simulink model "leg"  (R2014a)
settings: Solver=FixedStepDiscrete  StartTime=0.0  StopTime=inf  FixedStep=0.001  RelTol=1e-3
libraries: xpcethercatlib x35, simulink x29, slrtlib x11
settings Model: xpc_rtwmakecfg_data=_xpcethercatlib_  SimulationMode=external  BufferReuse=off  Creator=drl  LastModifiedBy=drl
settings SolverCC: EnableConcurrentExecution=on  ConcurrentTasks=on
settings OptimizationCC: BlockReduction=off  OptimizeBlockIOStorage=off  BufferReuse=off  GlobalBufferReuse=off  ExpressionFolding=off  LocalBlockOutputs=off
settings HardwareCC: ProdIntDivRoundTo=Zero  ProdEndianess=LittleEndian  ProdHWDeviceType=Generic->32-bit x86 compatible
settings RTWCC: SystemTargetFile=slrt.tlc  TemplateMakefile=slrt_default_tmf  Description=Simulink Real-Time  ProcessScript=slrt_make_rtw_hook  RTWCompilerOptimization=On
settings SimulinkRealTimeCC: GeneratePreprocessorConditionals=Disable all  EnableShiftOperators=on

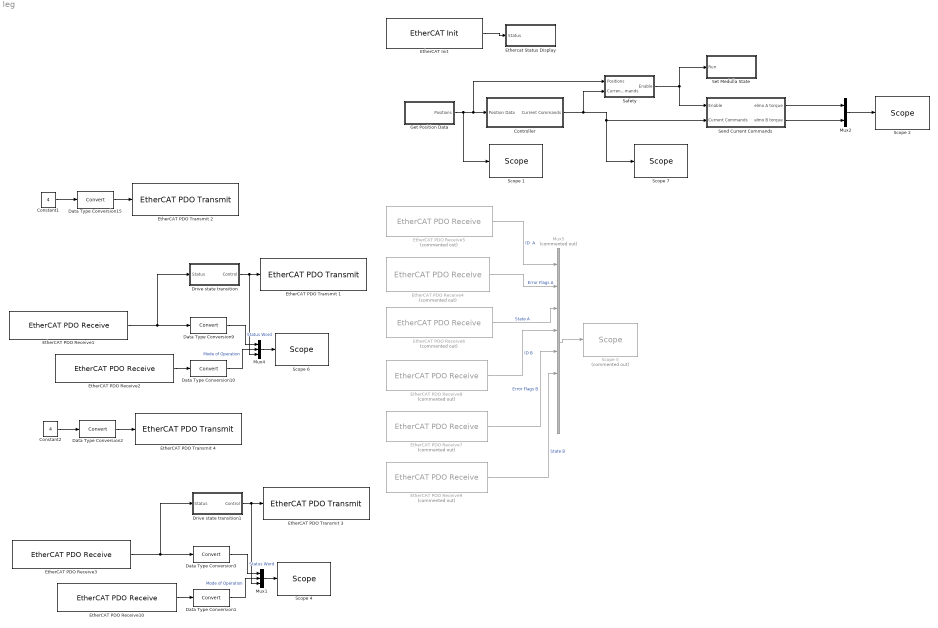
== system leg ==
  Constant1 : Constant  Value=4  OutDataTypeStr=Inherit: Inherit via back propagation  SampleTime=-1
  Constant2 : Constant  Value=4  OutDataTypeStr=Inherit: Inherit via back propagation  SampleTime=-1
  Controller : Subsystem
  Data Type Conversion{1..3,9..10,15} (6 alike) : DataTypeConversion
  Drive state transition : Subsystem
  Drive state transition1 : Subsystem
  "EtherCAT Init " : xpcethercatlib/EtherCAT Init   Priority=0  config_file=C:\Users\drl\Documents\MATLAB\2 medulla 2 elmo.xml  device_id=0  pci_bus=4  pci_slot=0  enaDebug=off  enaDC=on  errLink=off  masterDbg=off  stateChgDbg=off  baseClock=off  masterCfg=off  logFile='c:\dbglog.txt'  sample_time=0.001000
  EtherCAT PDO Receive1 : xpcethercatlib/EtherCAT PDO Receive  Priority=2  sig_name=Drive 1 (Elmo Drive).Inputs.Status word  sig_offset=1488  sig_type=uint16  type_size=16  sig_dim=1  device_id=0  sample_time=0.001000
  EtherCAT PDO Receive10 : xpcethercatlib/EtherCAT PDO Receive  Priority=2  sig_name=Drive 2 (Elmo Drive).Inputs.Mode of operation display  sig_offset=1584  sig_type=int8  type_size=8  sig_dim=1  device_id=0  sample_time=0.001000
  EtherCAT PDO Receive2 : xpcethercatlib/EtherCAT PDO Receive  Priority=2  sig_name=Drive 1 (Elmo Drive).Inputs.Mode of operation display  sig_offset=1504  sig_type=int8  type_size=8  sig_dim=1  device_id=0  sample_time=0.001000
  EtherCAT PDO Receive3 : xpcethercatlib/EtherCAT PDO Receive  Priority=2  sig_name=Drive 2 (Elmo Drive).Inputs.Status word  sig_offset=1568  sig_type=uint16  type_size=16  sig_dim=1  device_id=0  sample_time=0.001000
  EtherCAT PDO Receive4 : xpcethercatlib/EtherCAT PDO Receive  Priority=2  Commented=on  sig_name=Box 2 (ATRIAS 2.1 Leg (Medulla 1.5)).uController Status.Error Flags  sig_offset=616  sig_type=uint8  type_size=8  sig_dim=1  device_id=0  sample_time=0.001000
  EtherCAT PDO Receive5 : xpcethercatlib/EtherCAT PDO Receive  Priority=2  Commented=on  sig_name=Box 2 (ATRIAS 2.1 Leg (Medulla 1.5)).uController Status.ID  sig_offset=592  sig_type=uint8  type_size=8  sig_dim=1  device_id=0  sample_time=0.001000
  EtherCAT PDO Receive6 : xpcethercatlib/EtherCAT PDO Receive  Priority=2  Commented=on  sig_name=Box 2 (ATRIAS 2.1 Leg (Medulla 1.5)).uController Status.State  sig_offset=600  sig_type=uint8  type_size=8  sig_dim=1  device_id=0  sample_time=0.001000
  EtherCAT PDO Receive7 : xpcethercatlib/EtherCAT PDO Receive  Priority=2  Commented=on  sig_name=Box 3 (ATRIAS 2.1 Leg (Medulla 1.5)).uController Status.Error Flags  sig_offset=992  sig_type=uint8  type_size=8  sig_dim=1  device_id=0  sample_time=0.001000
  EtherCAT PDO Receive8 : xpcethercatlib/EtherCAT PDO Receive  Priority=2  Commented=on  sig_name=Box 3 (ATRIAS 2.1 Leg (Medulla 1.5)).uController Status.ID  sig_offset=968  sig_type=uint8  type_size=8  sig_dim=1  device_id=0  sample_time=0.001000
  EtherCAT PDO Receive9 : xpcethercatlib/EtherCAT PDO Receive  Priority=2  Commented=on  sig_name=Box 3 (ATRIAS 2.1 Leg (Medulla 1.5)).uController Status.State  sig_offset=976  sig_type=uint8  type_size=8  sig_dim=1  device_id=0  sample_time=0.001000
  EtherCAT PDO Transmit 1 : xpcethercatlib/EtherCAT PDO Transmit   Priority=3  sig_name=Drive 1 (Elmo Drive).Outputs.Control word  sig_offset=1456  sig_type=uint16  type_size=16  sig_dim=1  device_id=0  sample_time=0.001000
  EtherCAT PDO Transmit 2 : xpcethercatlib/EtherCAT PDO Transmit   Priority=3  sig_name=Drive 1 (Elmo Drive).Outputs.Mode of operation  sig_offset=1472  sig_type=int8  type_size=8  sig_dim=1  device_id=0  sample_time=0.001000
  EtherCAT PDO Transmit 3 : xpcethercatlib/EtherCAT PDO Transmit   Priority=3  sig_name=Drive 2 (Elmo Drive).Outputs.Control word  sig_offset=1536  sig_type=uint16  type_size=16  sig_dim=1  device_id=0  sample_time=0.001000
  EtherCAT PDO Transmit 4 : xpcethercatlib/EtherCAT PDO Transmit   Priority=3  sig_name=Drive 2 (Elmo Drive).Outputs.Mode of operation  sig_offset=1552  sig_type=int8  type_size=8  sig_dim=1  device_id=0  sample_time=0.001000
  Ethercat Status Display : Subsystem
  Get Position Data : Subsystem
  Mux1 : Mux  Inputs=3
  Mux2 : Mux  Inputs=2
  Mux4 : Mux  Inputs=3
  Mux5 : Mux  Commented=on  Inputs=8
  Safety : Subsystem
  Scope 1 : slrtlib/Displays and Logging/Scope   scopeno=3  scopetype=Target  autostart=on  viewmode=Numerical  formatstr='%15.6f'  grid=on  ylimits=[0,0]  nosamples=100  noprepostsamples=0  interleave=1  triggermode=FreeRun  triggersignal=1  trigsignalfromport=off  triggerlevel=0.0  triggerslope=Either  triggerscope=1  triggersample=0  filename=data.dat  mode=Lazy  writesize=512  autorestart=off  dynamicfilemode=off  maxwritefilesize=512*1024^2
  Scope 2 : slrtlib/Displays and Logging/Scope   scopeno=4  scopetype=Target  autostart=on  viewmode=Numerical  formatstr='%15.6f'  grid=on  ylimits=[0,0]  nosamples=100  noprepostsamples=0  interleave=1  triggermode=FreeRun  triggersignal=1  trigsignalfromport=off  triggerlevel=0.0  triggerslope=Either  triggerscope=1  triggersample=0  filename=data.dat  mode=Lazy  writesize=512  autorestart=off  dynamicfilemode=off  maxwritefilesize=512*1024^2
  Scope 4 : slrtlib/Displays and Logging/Scope   scopeno=5  scopetype=Target  autostart=on  viewmode=Numerical  formatstr='%f'  grid=on  ylimits=[0,0]  nosamples=100  noprepostsamples=0  interleave=1  triggermode=FreeRun  triggersignal=1  trigsignalfromport=off  triggerlevel=0.0  triggerslope=Either  triggerscope=2  triggersample=0  filename=data.dat  mode=Lazy  writesize=512  autorestart=off  dynamicfilemode=off  maxwritefilesize=512*1024^2
  Scope 5 : slrtlib/Displays and Logging/Scope   Commented=on  scopeno=5  scopetype=Target  autostart=on  viewmode=Numerical  formatstr='%15.6f'  grid=on  ylimits=[0,0]  nosamples=100  noprepostsamples=0  interleave=1  triggermode=FreeRun  triggersignal=1  trigsignalfromport=off  triggerlevel=0.0  triggerslope=Either  triggerscope=1  triggersample=0  filename=data.dat  mode=Lazy  writesize=512  autorestart=off  dynamicfilemode=off  maxwritefilesize=512*1024^2
  Scope 6 : slrtlib/Displays and Logging/Scope   scopeno=10  scopetype=Target  autostart=on  viewmode=Numerical  formatstr='%f'  grid=on  ylimits=[0,0]  nosamples=100  noprepostsamples=0  interleave=1  triggermode=FreeRun  triggersignal=1  trigsignalfromport=off  triggerlevel=0.0  triggerslope=Either  triggerscope=2  triggersample=0  filename=data.dat  mode=Lazy  writesize=512  autorestart=off  dynamicfilemode=off  maxwritefilesize=512*1024^2
  Scope 7 : slrtlib/Displays and Logging/Scope   scopeno=7  scopetype=Target  autostart=on  viewmode=Numerical  formatstr='%15.6f'  grid=on  ylimits=[0,0]  nosamples=100  noprepostsamples=0  interleave=1  triggermode=FreeRun  triggersignal=1  trigsignalfromport=off  triggerlevel=0.0  triggerslope=Either  triggerscope=1  triggersample=0  filename=data.dat  mode=Lazy  writesize=512  autorestart=off  dynamicfilemode=off  maxwritefilesize=512*1024^2
  Send Current Commands : Subsystem
  Set Medulla State : Subsystem
  wires:
  Mux5/1 -> Scope 5/1
  EtherCAT PDO Receive5/1 -> Mux5/1  "ID  A"
  EtherCAT PDO Receive4/1 -> Mux5/2  "Error Flags A"
  EtherCAT PDO Receive6/1 -> Mux5/3  "State A"
  EtherCAT PDO Receive8/1 -> Mux5/4  "ID B"
  EtherCAT PDO Receive7/1 -> Mux5/5  "Error Flags B"
  EtherCAT PDO Receive9/1 -> Mux5/6  "State B"
  Get Position Data/1("Positions ") -> Safety/1(Positions), Controller/1(Position Data), Scope 1/1
  Controller/1(Current Commands) -> Safety/2(Current Commands), Send Current Commands/2(Current Commands), Scope 7/1
  Safety/1(Enable) -> Set Medulla State/1(Run), Send Current Commands/1(Enable)
  "EtherCAT Init "/1 -> Ethercat Status Display/1(Status)
  EtherCAT PDO Receive1/1 -> Drive state transition/1(Status), Data Type Conversion9/1
  EtherCAT PDO Receive2/1 -> Data Type Conversion10/1
  Mux4/1 -> Scope 6/1
  Data Type Conversion9/1 -> Mux4/1  "Status Word"
  Data Type Conversion10/1 -> Mux4/2  "Mode of Operation"
  Constant1/1 -> Data Type Conversion15/1
  Drive state transition/1(Control) -> Mux4/3, EtherCAT PDO Transmit 1/1
  Data Type Conversion15/1 -> EtherCAT PDO Transmit 2/1
  Send Current Commands/1(elmo A torque) -> Mux2/1
  Send Current Commands/2(elmo B torque) -> Mux2/2
  EtherCAT PDO Receive3/1 -> Drive state transition1/1(Status), Data Type Conversion3/1
  EtherCAT PDO Receive10/1 -> Data Type Conversion1/1
  Mux1/1 -> Scope 4/1
  Data Type Conversion3/1 -> Mux1/1  "Status Word"
  Data Type Conversion1/1 -> Mux1/2  "Mode of Operation"
  Constant2/1 -> Data Type Conversion2/1
  Drive state transition1/1(Control) -> Mux1/3, EtherCAT PDO Transmit 3/1
  Data Type Conversion2/1 -> EtherCAT PDO Transmit 4/1
  Mux2/1 -> Scope 2/1

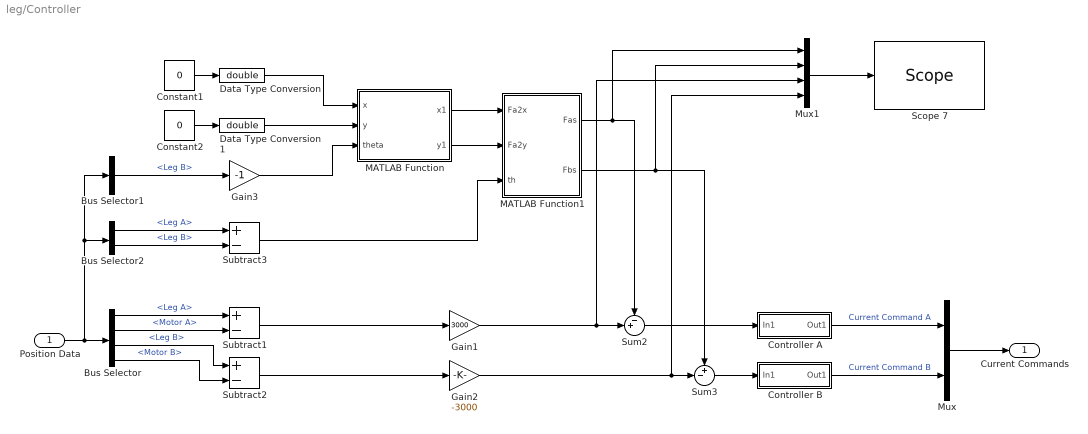
== system leg/Controller ==
  Position Data : Inport
  Bus Selector : BusSelector  OutputSignals=Leg A,Motor A,Leg B,Motor B
  Bus Selector1 : BusSelector  OutputSignals=Leg B
  Bus Selector2 : BusSelector  OutputSignals=Leg A,Leg B
  Constant1 : Constant  Value=0
  Constant2 : Constant  Value=0
  Controller A : Subsystem
  Controller B : Subsystem
  Data Type Conversion : DataTypeConversion  OutDataTypeStr=double
  Data Type Conversion1 : DataTypeConversion  OutDataTypeStr=double
  Gain1 : Gain  Gain=3000
  Gain2 : Gain  Gain=-3000
  Gain3 : Gain  Gain=-1
  MATLAB Function : MATLAB Function  TreatAsAtomicUnit=on
  MATLAB Function1 : MATLAB Function  TreatAsAtomicUnit=on
  Mux : Mux  Inputs=2
  Mux1 : Mux
  Scope 7 : slrtlib/Displays and Logging/Scope   scopeno=9  scopetype=Target  autostart=on  viewmode=Numerical  formatstr='%15.6f'  grid=on  ylimits=[0,0]  nosamples=100  noprepostsamples=0  interleave=1  triggermode=FreeRun  triggersignal=1  trigsignalfromport=off  triggerlevel=0.0  triggerslope=Either  triggerscope=1  triggersample=0  filename=data.dat  mode=Lazy  writesize=512  autorestart=off  dynamicfilemode=off  maxwritefilesize=512*1024^2
  Subtract1 : Sum  Inputs=+-
  Subtract2 : Sum  Inputs=+-
  Subtract3 : Sum  Inputs=+-
  Sum2 : Sum  Inputs=-+|
  Sum3 : Sum  Inputs=+-|
  Current Commands : Outport
  wires:
  Position Data/1 -> Bus Selector1/1, Bus Selector2/1, Bus Selector/1
  Mux1/1 -> Scope 7/1
  Bus Selector/4 -> Subtract2/2  "<Motor B>"
  Bus Selector/1 -> Subtract1/1  "<Leg A>"
  Bus Selector/2 -> Subtract1/2  "<Motor A>"
  Bus Selector/3 -> Subtract2/1  "<Leg B>"
  Subtract2/1 -> Gain2/1
  Subtract1/1 -> Gain1/1
  Gain2/1 -> Mux1/4, Sum3/2
  Gain1/1 -> Sum2/2, Mux1/3
  MATLAB Function/1(x1) -> MATLAB Function1/1(Fa2x)
  MATLAB Function/2(y1) -> MATLAB Function1/2(Fa2y)
  Bus Selector2/1 -> Subtract3/1  "<Leg A>"
  Bus Selector2/2 -> Subtract3/2  "<Leg B>"
  MATLAB Function1/1(Fas) -> Mux1/1, Sum2/1
  MATLAB Function1/2(Fbs) -> Sum3/1, Mux1/2
  Sum3/1 -> Controller B/1(In1)
  Sum2/1 -> Controller A/1(In1)
  Mux/1 -> Current Commands/1
  Controller A/1(Out1) -> Mux/1  "Current Command A"
  Controller B/1(Out1) -> Mux/2  "Current Command B"
  Bus Selector1/1 -> Gain3/1  "<Leg B>"
  Gain3/1 -> MATLAB Function/3(theta)
  Data Type Conversion1/1 -> MATLAB Function/2(y)
  Constant2/1 -> Data Type Conversion1/1
  Constant1/1 -> Data Type Conversion/1
  Data Type Conversion/1 -> MATLAB Function/1(x)
  Subtract3/1 -> MATLAB Function1/3(th)

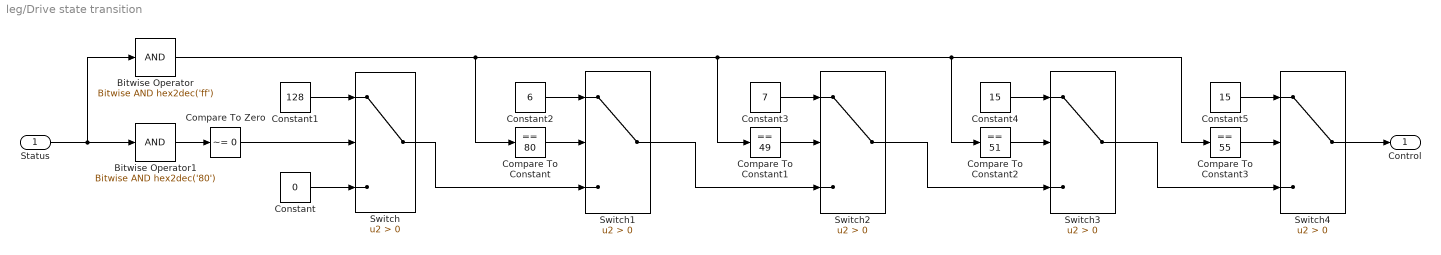
== system leg/Drive state transition ==
  Status : Inport
  Bitwise Operator : simulink/Logic and Bit Operations/Bitwise Operator  logicop=AND  UseBitMask=on  BitMask=hex2dec('ff')  BitMaskRealWorld=Stored Integer
  Bitwise Operator1 : simulink/Logic and Bit Operations/Bitwise Operator  logicop=AND  UseBitMask=on  BitMask=hex2dec('80')  BitMaskRealWorld=Stored Integer
  Compare To Constant : simulink/Logic and Bit Operations/Compare To Constant  relop===  const=80  OutDataTypeStr=boolean
  Compare To Constant1 : simulink/Logic and Bit Operations/Compare To Constant  relop===  const=49  OutDataTypeStr=boolean
  Compare To Constant2 : simulink/Logic and Bit Operations/Compare To Constant  relop===  const=51  OutDataTypeStr=boolean
  Compare To Constant3 : simulink/Logic and Bit Operations/Compare To Constant  relop===  const=55  OutDataTypeStr=boolean
  Compare To Zero : simulink/Logic and Bit Operations/Compare To Zero  relop=~=  OutDataTypeStr=boolean
  Constant : Constant  Value=0  OutDataTypeStr=uint16
  Constant1 : Constant  Value=128  OutDataTypeStr=uint16
  Constant2 : Constant  Value=6  OutDataTypeStr=uint16
  Constant3 : Constant  Value=7  OutDataTypeStr=uint16
  Constant4 : Constant  Value=15  OutDataTypeStr=uint16
  Constant5 : Constant  Value=15  OutDataTypeStr=uint16
  Switch{,1..4} (5 alike) : Switch  Criteria=u2 > Threshold
  Control : Outport
  wires:
  Status/1 -> Bitwise Operator/1, Bitwise Operator1/1
  Bitwise Operator1/1 -> Compare To Zero/1
  Compare To Zero/1 -> Switch/2
  Constant1/1 -> Switch/1
  Constant/1 -> Switch/3
  Compare To Constant/1 -> Switch1/2
  Switch/1 -> Switch1/3
  Bitwise Operator/1 -> Compare To Constant3/1, Compare To Constant2/1, Compare To Constant1/1, Compare To Constant/1
  Constant2/1 -> Switch1/1
  Compare To Constant1/1 -> Switch2/2
  Switch1/1 -> Switch2/3
  Constant3/1 -> Switch2/1
  Compare To Constant2/1 -> Switch3/2
  Switch2/1 -> Switch3/3
  Constant4/1 -> Switch3/1
  Compare To Constant3/1 -> Switch4/2
  Switch3/1 -> Switch4/3
  Constant5/1 -> Switch4/1
  Switch4/1 -> Control/1

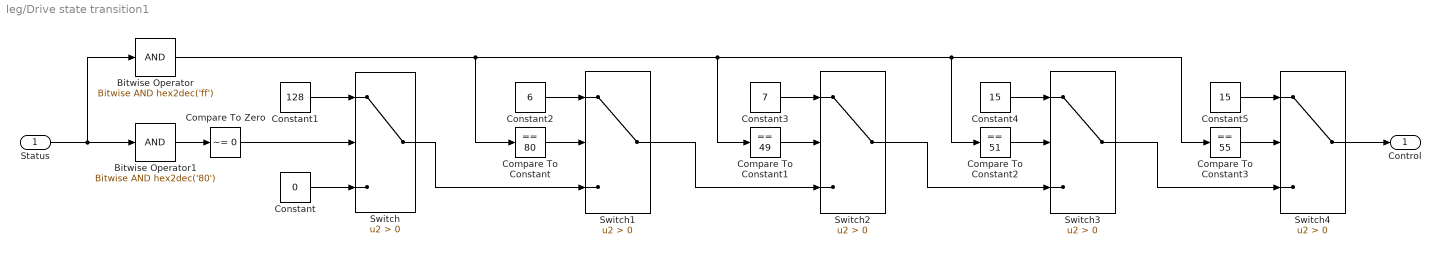
== system leg/Drive state transition1 ==
  Status : Inport
  Bitwise Operator : simulink/Logic and Bit Operations/Bitwise Operator  logicop=AND  UseBitMask=on  BitMask=hex2dec('ff')  BitMaskRealWorld=Stored Integer
  Bitwise Operator1 : simulink/Logic and Bit Operations/Bitwise Operator  logicop=AND  UseBitMask=on  BitMask=hex2dec('80')  BitMaskRealWorld=Stored Integer
  Compare To Constant : simulink/Logic and Bit Operations/Compare To Constant  relop===  const=80  OutDataTypeStr=boolean
  Compare To Constant1 : simulink/Logic and Bit Operations/Compare To Constant  relop===  const=49  OutDataTypeStr=boolean
  Compare To Constant2 : simulink/Logic and Bit Operations/Compare To Constant  relop===  const=51  OutDataTypeStr=boolean
  Compare To Constant3 : simulink/Logic and Bit Operations/Compare To Constant  relop===  const=55  OutDataTypeStr=boolean
  Compare To Zero : simulink/Logic and Bit Operations/Compare To Zero  relop=~=  OutDataTypeStr=boolean
  Constant : Constant  Value=0  OutDataTypeStr=uint16
  Constant1 : Constant  Value=128  OutDataTypeStr=uint16
  Constant2 : Constant  Value=6  OutDataTypeStr=uint16
  Constant3 : Constant  Value=7  OutDataTypeStr=uint16
  Constant4 : Constant  Value=15  OutDataTypeStr=uint16
  Constant5 : Constant  Value=15  OutDataTypeStr=uint16
  Switch{,1..4} (5 alike) : Switch  Criteria=u2 > Threshold
  Control : Outport
  wires:
  Status/1 -> Bitwise Operator/1, Bitwise Operator1/1
  Bitwise Operator1/1 -> Compare To Zero/1
  Compare To Zero/1 -> Switch/2
  Constant1/1 -> Switch/1
  Constant/1 -> Switch/3
  Compare To Constant/1 -> Switch1/2
  Switch/1 -> Switch1/3
  Bitwise Operator/1 -> Compare To Constant3/1, Compare To Constant2/1, Compare To Constant1/1, Compare To Constant/1
  Constant2/1 -> Switch1/1
  Compare To Constant1/1 -> Switch2/2
  Switch1/1 -> Switch2/3
  Constant3/1 -> Switch2/1
  Compare To Constant2/1 -> Switch3/2
  Switch2/1 -> Switch3/3
  Constant4/1 -> Switch3/1
  Compare To Constant3/1 -> Switch4/2
  Switch3/1 -> Switch4/3
  Constant5/1 -> Switch4/1
  Switch4/1 -> Control/1

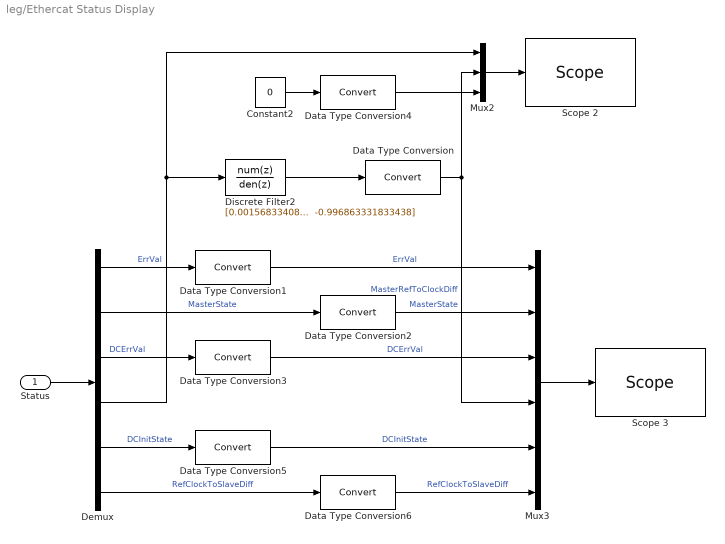
== system leg/Ethercat Status Display ==
  Status : Inport
  Constant2 : Constant  Value=0  OutDataTypeStr=Inherit: Inherit via back propagation  SampleTime=-1
  Data Type Conversion{,1..6} (7 alike) : DataTypeConversion
  Demux : Demux  Outputs=6
  Discrete Filter2 : DiscreteFilter  Numerator="[0.001568334083281   0.001568334083281]"  Denominator="[1.000000000000000  -0.996863331833438]"  a0EqualsOne=on
  Mux2 : Mux  Inputs=3
  Mux3 : Mux  Inputs=6
  Scope 2 : slrtlib/Displays and Logging/Scope   scopeno=6  scopetype=Target  autostart=on  viewmode=Graphical rolling  formatstr='%f'  grid=on  ylimits=[0,0]  nosamples=10000  noprepostsamples=0  interleave=1  triggermode=FreeRun  triggersignal=1  trigsignalfromport=off  triggerlevel=0.0  triggerslope=Either  triggerscope=1  triggersample=0  filename=data.dat  mode=Lazy  writesize=512  autorestart=off  dynamicfilemode=off  maxwritefilesize=512*1024^2
  Scope 3 : slrtlib/Displays and Logging/Scope   scopeno=2  scopetype=Target  autostart=on  viewmode=Numerical  formatstr='%15.6f'  grid=on  ylimits=[0,0]  nosamples=100  noprepostsamples=0  interleave=1  triggermode=FreeRun  triggersignal=1  trigsignalfromport=off  triggerlevel=0.0  triggerslope=Either  triggerscope=1  triggersample=0  filename=data.dat  mode=Lazy  writesize=512  autorestart=off  dynamicfilemode=off  maxwritefilesize=512*1024^2
  wires:
  Status/1 -> Demux/1
  Demux/4 -> Discrete Filter2/1, Mux2/1
  Discrete Filter2/1 -> Data Type Conversion/1
  Mux2/1 -> Scope 2/1
  Constant2/1 -> Data Type Conversion4/1
  Data Type Conversion4/1 -> Mux2/3
  Mux3/1 -> Scope 3/1
  Data Type Conversion/1 -> Mux3/4, Mux2/2  "MasterRefToClockDiff"
  Data Type Conversion1/1 -> Mux3/1  "ErrVal"
  Data Type Conversion2/1 -> Mux3/2  "MasterState"
  Data Type Conversion3/1 -> Mux3/3  "DCErrVal"
  Data Type Conversion5/1 -> Mux3/5  "DCInitState"
  Data Type Conversion6/1 -> Mux3/6  "RefClockToSlaveDiff"
  Demux/1 -> Data Type Conversion1/1  "ErrVal"
  Demux/2 -> Data Type Conversion2/1  "MasterState"
  Demux/3 -> Data Type Conversion3/1  "DCErrVal"
  Demux/5 -> Data Type Conversion5/1  "DCInitState"
  Demux/6 -> Data Type Conversion6/1  "RefClockToSlaveDiff"

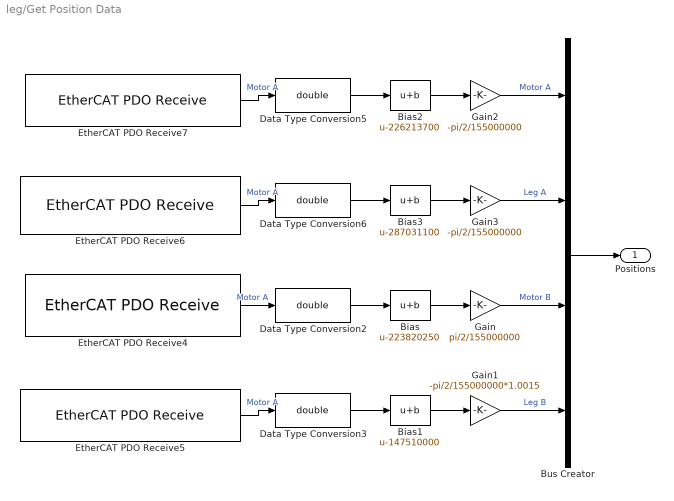
== system leg/Get Position Data ==
  Bias : Bias  Bias=-223820250
  Bias1 : Bias  Bias=-147510000
  Bias2 : Bias  Bias=-226213700
  Bias3 : Bias  Bias=-287031100
  Bus Creator : BusCreator
  Data Type Conversion{2..3,5..6} (4 alike) : DataTypeConversion  OutDataTypeStr=double
  EtherCAT PDO Receive4 : xpcethercatlib/EtherCAT PDO Receive  Priority=2  sig_name=Box 3 (ATRIAS 2.1 Leg (Medulla 1.5)).Motor Encoder.Motor Encoder  sig_offset=648  sig_type=uint32  type_size=32  sig_dim=1  device_id=0  sample_time=0.001000
  EtherCAT PDO Receive5 : xpcethercatlib/EtherCAT PDO Receive  Priority=2  sig_name=Box 3 (ATRIAS 2.1 Leg (Medulla 1.5)).Leg Encoder.Leg Encoder  sig_offset=696  sig_type=uint32  type_size=32  sig_dim=1  device_id=0  sample_time=0.001000
  EtherCAT PDO Receive6 : xpcethercatlib/EtherCAT PDO Receive  Priority=2  sig_name=Box 4 (ATRIAS 2.1 Leg (Medulla 1.5)).Leg Encoder.Leg Encoder  sig_offset=1072  sig_type=uint32  type_size=32  sig_dim=1  device_id=0  sample_time=0.001000
  EtherCAT PDO Receive7 : xpcethercatlib/EtherCAT PDO Receive  Priority=2  sig_name=Box 4 (ATRIAS 2.1 Leg (Medulla 1.5)).Motor Encoder.Motor Encoder  sig_offset=1024  sig_type=uint32  type_size=32  sig_dim=1  device_id=0  sample_time=0.001000
  Gain : Gain  Gain=pi/2/155000000
  Gain1 : Gain  Gain=-pi/2/155000000*1.0015
  Gain2 : Gain  Gain=-pi/2/155000000
  Gain3 : Gain  Gain=-pi/2/155000000
  "Positions " : Outport
  wires:
  Gain/1 -> Bus Creator/3  "Motor B"
  Gain1/1 -> Bus Creator/4  "Leg B"
  Gain2/1 -> Bus Creator/1  "Motor A"
  Gain3/1 -> Bus Creator/2  "Leg A"
  EtherCAT PDO Receive4/1 -> Data Type Conversion2/1  "Motor A"
  Data Type Conversion2/1 -> Bias/1
  Bias/1 -> Gain/1
  EtherCAT PDO Receive5/1 -> Data Type Conversion3/1  "Motor A"
  Data Type Conversion3/1 -> Bias1/1
  Bias1/1 -> Gain1/1
  EtherCAT PDO Receive7/1 -> Data Type Conversion5/1  "Motor A"
  Data Type Conversion5/1 -> Bias2/1
  Bias2/1 -> Gain2/1
  EtherCAT PDO Receive6/1 -> Data Type Conversion6/1  "Motor A"
  Data Type Conversion6/1 -> Bias3/1
  Bias3/1 -> Gain3/1
  Bus Creator/1 -> "Positions "/1

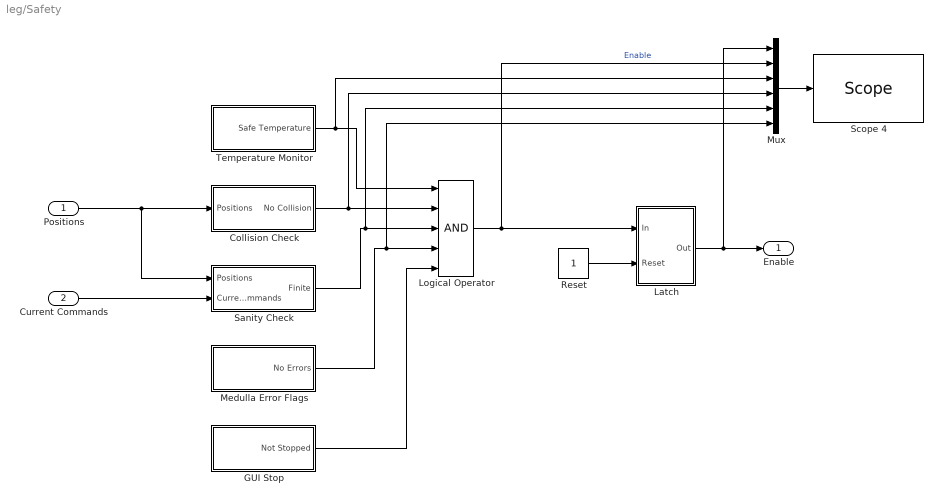
== system leg/Safety ==
  Positions : Inport
  Current Commands : Inport  Port=2
  Collision Check : Subsystem
  GUI Stop : Subsystem
  Latch : Subsystem
  Logical Operator : Logic  Inputs=5  AllPortsSameDT=off  OutDataTypeStr=boolean
  Medulla Error Flags : Subsystem
  Mux : Mux  Inputs=6
  Reset : Constant
  Sanity Check : Subsystem
  Scope 4 : slrtlib/Displays and Logging/Scope   scopeno=1  scopetype=Target  autostart=on  viewmode=Numerical  formatstr='%15.6f'  grid=on  ylimits=[0,0]  nosamples=100  noprepostsamples=0  interleave=1  triggermode=FreeRun  triggersignal=1  trigsignalfromport=off  triggerlevel=0.0  triggerslope=Either  triggerscope=1  triggersample=0  filename=data.dat  mode=Lazy  writesize=512  autorestart=off  dynamicfilemode=off  maxwritefilesize=512*1024^2
  Temperature Monitor : Subsystem
  Enable : Outport
  wires:
  Collision Check/1(No Collision) -> Mux/4, Logical Operator/2
  Temperature Monitor/1(Safe Temperature) -> Mux/3, Logical Operator/1
  Positions/1 -> Sanity Check/1(Positions), Collision Check/1(Positions)
  Latch/1(Out) -> Mux/1, Enable/1
  Current Commands/1 -> Sanity Check/2(Current Commands)
  Sanity Check/1(Finite) -> Mux/5, Logical Operator/3
  Logical Operator/1 -> Mux/2, Latch/1(In)  "Enable"
  Reset/1 -> Latch/2(Reset)
  Medulla Error Flags/1(No Errors) -> Mux/6, Logical Operator/4
  Mux/1 -> Scope 4/1
  GUI Stop/1(Not Stopped) -> Logical Operator/5

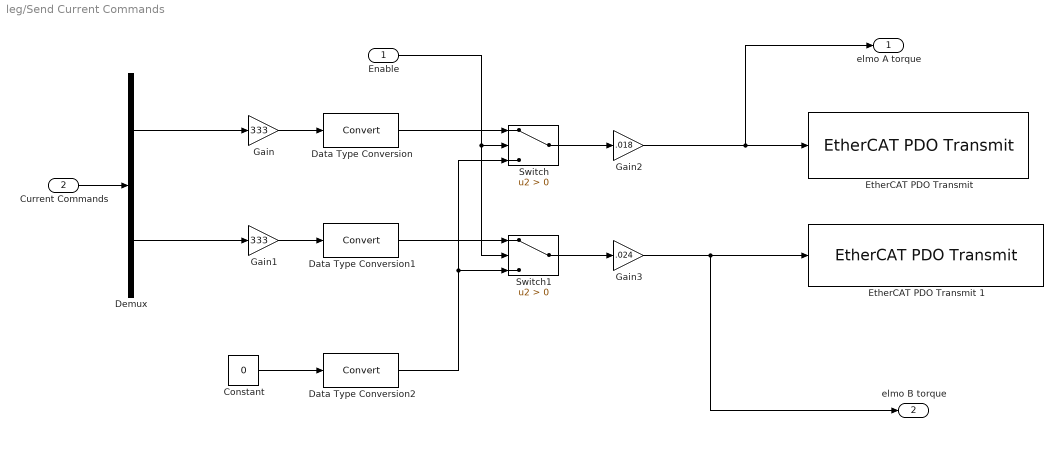
== system leg/Send Current Commands ==
  Enable : Inport
  Current Commands : Inport  Port=2
  Constant : Constant  Value=0  SampleTime=-1
  Data Type Conversion : DataTypeConversion
  Data Type Conversion1 : DataTypeConversion
  Data Type Conversion2 : DataTypeConversion
  Demux : Demux  Outputs=2
  "EtherCAT PDO Transmit " : xpcethercatlib/EtherCAT PDO Transmit   Priority=3  sig_name=Drive 1 (Elmo Drive).Outputs.Target Torque  sig_offset=1440  sig_type=int16  type_size=16  sig_dim=1  device_id=0  sample_time=0.001000
  EtherCAT PDO Transmit 1 : xpcethercatlib/EtherCAT PDO Transmit   Priority=3  sig_name=Drive 2 (Elmo Drive).Outputs.Target Torque  sig_offset=1520  sig_type=int16  type_size=16  sig_dim=1  device_id=0  sample_time=0.001000
  Gain : Gain  Gain=333
  Gain1 : Gain  Gain=333
  Gain2 : Gain  Gain=.018  OutDataTypeStr=int16
  Gain3 : Gain  Gain=.024  OutDataTypeStr=int16
  Switch : Switch  Criteria=u2 > Threshold  OutDataTypeStr=int16
  Switch1 : Switch  Criteria=u2 > Threshold  OutDataTypeStr=int16
  elmo A torque : Outport
  elmo B torque : Outport  Port=2
  wires:
  Data Type Conversion1/1 -> Switch1/1
  Data Type Conversion/1 -> Switch/1
  Enable/1 -> Switch/2, Switch1/2
  Data Type Conversion2/1 -> Switch/3, Switch1/3
  Constant/1 -> Data Type Conversion2/1
  Gain/1 -> Data Type Conversion/1
  Gain1/1 -> Data Type Conversion1/1
  Current Commands/1 -> Demux/1
  Demux/2 -> Gain1/1
  Demux/1 -> Gain/1
  Gain2/1 -> "EtherCAT PDO Transmit "/1, elmo A torque/1
  Switch/1 -> Gain2/1
  Switch1/1 -> Gain3/1
  Gain3/1 -> EtherCAT PDO Transmit 1/1, elmo B torque/1

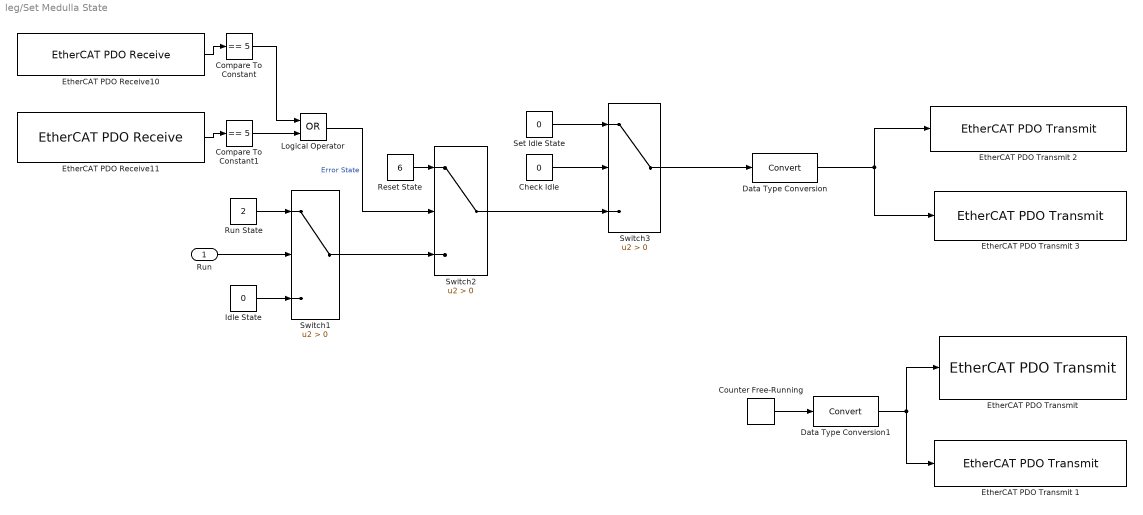
== system leg/Set Medulla State ==
  Run : Inport
  Check Idle : Constant  Value=0
  Compare To Constant : simulink/Logic and Bit Operations/Compare To Constant  relop===  const=5  OutDataTypeStr=boolean
  Compare To Constant1 : simulink/Logic and Bit Operations/Compare To Constant  relop===  const=5  OutDataTypeStr=boolean
  Counter Free-Running : simulink/Sources/Counter Free-Running  NumBits=16  tsamp=-1
  Data Type Conversion : DataTypeConversion
  Data Type Conversion1 : DataTypeConversion
  EtherCAT PDO Receive10 : xpcethercatlib/EtherCAT PDO Receive  Priority=2  sig_name=Box 4 (ATRIAS 2.1 Leg (Medulla 1.5)).uController Status.State  sig_offset=976  sig_type=uint8  type_size=8  sig_dim=1  device_id=0  sample_time=0.001000
  EtherCAT PDO Receive11 : xpcethercatlib/EtherCAT PDO Receive  Priority=2  sig_name=Box 3 (ATRIAS 2.1 Leg (Medulla 1.5)).uController Status.State  sig_offset=600  sig_type=uint8  type_size=8  sig_dim=1  device_id=0  sample_time=0.001000
  "EtherCAT PDO Transmit " : xpcethercatlib/EtherCAT PDO Transmit   Priority=3  sig_name=Box 4 (ATRIAS 2.1 Leg (Medulla 1.5)).uControllerInput.Counter  sig_offset=976  sig_type=uint16  type_size=16  sig_dim=1  device_id=0  sample_time=0.001000
  EtherCAT PDO Transmit 1 : xpcethercatlib/EtherCAT PDO Transmit   Priority=3  sig_name=Box 3 (ATRIAS 2.1 Leg (Medulla 1.5)).uControllerInput.Counter  sig_offset=600  sig_type=uint16  type_size=16  sig_dim=1  device_id=0  sample_time=0.001000
  EtherCAT PDO Transmit 2 : xpcethercatlib/EtherCAT PDO Transmit   Priority=3  sig_name=Box 4 (ATRIAS 2.1 Leg (Medulla 1.5)).uControllerInput.Command  sig_offset=968  sig_type=uint8  type_size=8  sig_dim=1  device_id=0  sample_time=0.001000
  EtherCAT PDO Transmit 3 : xpcethercatlib/EtherCAT PDO Transmit   Priority=3  sig_name=Box 3 (ATRIAS 2.1 Leg (Medulla 1.5)).uControllerInput.Command  sig_offset=592  sig_type=uint8  type_size=8  sig_dim=1  device_id=0  sample_time=0.001000
  Idle State : Constant  Value=0
  Logical Operator : Logic  Operator=OR  AllPortsSameDT=off  OutDataTypeStr=boolean
  Reset State : Constant  Value=6
  Run State : Constant  Value=2
  Set Idle State : Constant  Value=0
  Switch1 : Switch  Criteria=u2 > Threshold
  Switch2 : Switch  Criteria=u2 > Threshold
  Switch3 : Switch  Criteria=u2 > Threshold
  wires:
  Data Type Conversion1/1 -> EtherCAT PDO Transmit 1/1, "EtherCAT PDO Transmit "/1
  Counter Free-Running/1 -> Data Type Conversion1/1
  Run/1 -> Switch1/2
  Run State/1 -> Switch1/1
  Idle State/1 -> Switch1/3
  Compare To Constant1/1 -> Logical Operator/2
  Compare To Constant/1 -> Logical Operator/1
  EtherCAT PDO Receive10/1 -> Compare To Constant/1
  EtherCAT PDO Receive11/1 -> Compare To Constant1/1
  Logical Operator/1 -> Switch2/2  "Error State"
  Switch1/1 -> Switch2/3
  Reset State/1 -> Switch2/1
  Switch2/1 -> Switch3/3
  Data Type Conversion/1 -> EtherCAT PDO Transmit 2/1, EtherCAT PDO Transmit 3/1
  Set Idle State/1 -> Switch3/1
  Switch3/1 -> Data Type Conversion/1
  Check Idle/1 -> Switch3/2

== system leg/Controller/Controller A ==
  In1 : Inport
  Discrete Derivative : simulink/Discrete/Discrete Derivative  gainval=1.0  ICPrevScaledInput=0.0  InputProcessing=Inherited  OutMin=[]  OutMax=[]  OutDataType=fixdt(1, 16)  OutScaling=2^-10  DoSatur=off
  Discrete Filter : DiscreteFilter  Numerator=[0.05 0.05]  Denominator=[1 0.9]  a0EqualsOne=on
  Kd : Gain  Gain=0.05
  Kp : Gain  Gain=2
  Saturation : Saturate  UpperLimit=15  LowerLimit=-15
  Sum : Sum  Inputs=|++
  Out1 : Outport
  wires:
  Discrete Derivative/1 -> Kd/1
  Kd/1 -> Sum/2
  Kp/1 -> Sum/1
  In1/1 -> Discrete Filter/1, Kp/1
  Saturation/1 -> Out1/1
  Sum/1 -> Saturation/1
  Discrete Filter/1 -> Discrete Derivative/1

== system leg/Controller/Controller B ==
  In1 : Inport
  Discrete Derivative : simulink/Discrete/Discrete Derivative  gainval=1.0  ICPrevScaledInput=0.0  InputProcessing=Inherited  OutMin=[]  OutMax=[]  OutDataType=fixdt(1, 16)  OutScaling=2^-10  DoSatur=off
  Discrete Filter : DiscreteFilter  Numerator=[0.05 0.05]  Denominator=[1 0.9]  a0EqualsOne=on
  Kd : Gain  Gain=0.05
  Kp : Gain  Gain=2
  Saturation : Saturate  UpperLimit=15  LowerLimit=-15
  Sum : Sum  Inputs=|++
  Out1 : Outport
  wires:
  Discrete Derivative/1 -> Kd/1
  Kd/1 -> Sum/2
  Kp/1 -> Sum/1
  In1/1 -> Discrete Filter/1, Kp/1
  Saturation/1 -> Out1/1
  Sum/1 -> Saturation/1
  Discrete Filter/1 -> Discrete Derivative/1

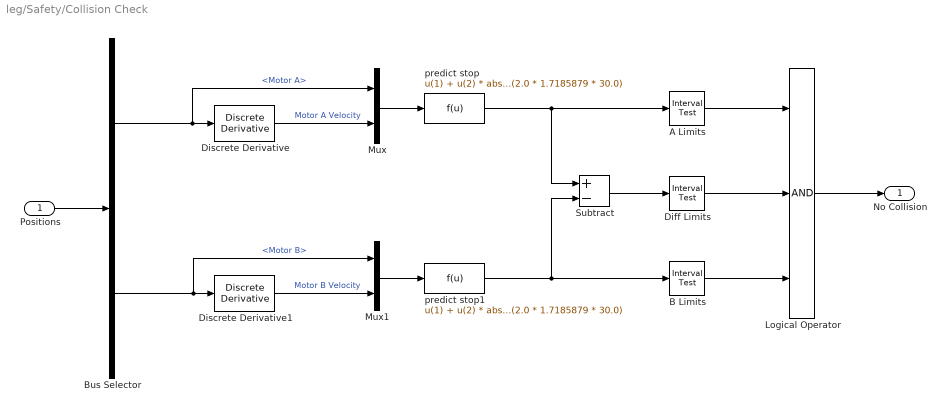
== system leg/Safety/Collision Check ==
  Positions : Inport
  A Limits : simulink/Logic and Bit Operations/Interval Test  IntervalClosedRight=off  uplimit=105/180*pi  IntervalClosedLeft=off  lowlimit=-45/180*pi  OutDataTypeStr=boolean
  B Limits : simulink/Logic and Bit Operations/Interval Test  IntervalClosedRight=off  uplimit=45/180*pi  IntervalClosedLeft=off  lowlimit=-105/180*pi  OutDataTypeStr=boolean
  Bus Selector : BusSelector  OutputSignals=Motor A,Motor B
  Diff Limits : simulink/Logic and Bit Operations/Interval Test  IntervalClosedRight=off  uplimit=135/180*pi  IntervalClosedLeft=off  lowlimit=5/180*pi  OutDataTypeStr=boolean
  Discrete Derivative : simulink/Discrete/Discrete Derivative  gainval=1.0  ICPrevScaledInput=0.0  InputProcessing=Inherited  OutMin=[]  OutMax=[]  OutDataType=fixdt(1, 16)  OutScaling=2^-10  DoSatur=off
  Discrete Derivative1 : simulink/Discrete/Discrete Derivative  gainval=1.0  ICPrevScaledInput=0.0  InputProcessing=Inherited  OutMin=[]  OutMax=[]  OutDataType=fixdt(1, 16)  OutScaling=2^-10  DoSatur=off
  Logical Operator : Logic  Inputs=3  AllPortsSameDT=off  OutDataTypeStr=boolean
  Mux : Mux  Inputs=2
  Mux1 : Mux  Inputs=2
  Subtract : Sum  Inputs=+-
  predict stop : Fcn  Expr=u(1) + u(2) * abs(u(2)) / (2.0 * 1.7185879 * 30.0)
  predict stop1 : Fcn  Expr=u(1) + u(2) * abs(u(2)) / (2.0 * 1.7185879 * 30.0)
  No Collision : Outport
  wires:
  predict stop/1 -> Subtract/1, A Limits/1
  predict stop1/1 -> Subtract/2, B Limits/1
  A Limits/1 -> Logical Operator/1
  B Limits/1 -> Logical Operator/3
  Logical Operator/1 -> No Collision/1
  Diff Limits/1 -> Logical Operator/2
  Subtract/1 -> Diff Limits/1
  Bus Selector/1 -> Discrete Derivative/1, Mux/1  "<Motor A>"
  Bus Selector/2 -> Mux1/1, Discrete Derivative1/1  "<Motor B>"
  Mux/1 -> predict stop/1
  Mux1/1 -> predict stop1/1
  Discrete Derivative/1 -> Mux/2  "Motor A Velocity"
  Discrete Derivative1/1 -> Mux1/2  "Motor B Velocity"
  Positions/1 -> Bus Selector/1

== system leg/Safety/GUI Stop ==
  Compare To Zero : simulink/Logic and Bit Operations/Compare To Zero  relop===  OutDataTypeStr=boolean
  Stop : Constant  Value=0
  Not Stopped : Outport
  wires:
  Stop/1 -> Compare To Zero/1
  Compare To Zero/1 -> Not Stopped/1

== system leg/Safety/Latch ==
  In : Inport
  Reset : Inport  Port=2
  Constant : Constant  Value=0  OutDataTypeStr=boolean
  Delay : Delay  DelayLength=1  InitialCondition=0
  Switch : Switch  Criteria=u2 > Threshold
  Switch1 : Switch  Criteria=u2 > Threshold
  Out : Outport
  wires:
  Reset/1 -> Switch1/2
  Switch/1 -> Switch1/3
  In/1 -> Switch1/1, Switch/1
  Switch1/1 -> Out/1, Delay/1
  Constant/1 -> Switch/3
  Delay/1 -> Switch/2

== system leg/Safety/Medulla Error Flags ==
  Compare To Zero : simulink/Logic and Bit Operations/Compare To Zero  relop===  OutDataTypeStr=boolean
  Compare To Zero1 : simulink/Logic and Bit Operations/Compare To Zero  relop===  OutDataTypeStr=boolean
  Error Flags A : Gain
  Error Flags B : Gain
  EtherCAT PDO Receive : xpcethercatlib/EtherCAT PDO Receive  Priority=2  sig_name=Box 4 (ATRIAS 2.1 Leg (Medulla 1.5)).uController Status.Error Flags  sig_offset=992  sig_type=uint8  type_size=8  sig_dim=1  device_id=0  sample_time=0.001000
  EtherCAT PDO Receive1 : xpcethercatlib/EtherCAT PDO Receive  Priority=2  sig_name=Box 3 (ATRIAS 2.1 Leg (Medulla 1.5)).uController Status.Error Flags  sig_offset=616  sig_type=uint8  type_size=8  sig_dim=1  device_id=0  sample_time=0.001000
  Ignore Encoder Errors : simulink/Logic and Bit Operations/Bit Clear  iBit=5
  Ignore Encoder Errors1 : simulink/Logic and Bit Operations/Bit Clear  iBit=5
  Logical Operator : Logic  AllPortsSameDT=off  OutDataTypeStr=boolean
  No Errors : Outport
  wires:
  Compare To Zero/1 -> Logical Operator/1
  Compare To Zero1/1 -> Logical Operator/2
  Logical Operator/1 -> No Errors/1
  EtherCAT PDO Receive/1 -> Error Flags A/1
  Error Flags A/1 -> Ignore Encoder Errors/1
  EtherCAT PDO Receive1/1 -> Error Flags B/1
  Error Flags B/1 -> Ignore Encoder Errors1/1
  Ignore Encoder Errors/1 -> Compare To Zero/1
  Ignore Encoder Errors1/1 -> Compare To Zero1/1

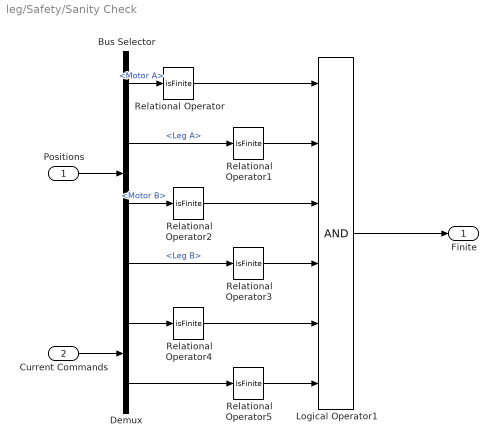
== system leg/Safety/Sanity Check ==
  Positions : Inport
  Current Commands : Inport  Port=2
  Bus Selector : BusSelector  OutputSignals=Motor A,Leg A,Motor B,Leg B
  Demux : Demux  Outputs=2
  Logical Operator1 : Logic  Inputs=6  AllPortsSameDT=off  OutDataTypeStr=boolean
  Relational Operator{,1..5} (6 alike) : RelationalOperator  Operator=isFinite  OutDataTypeStr=boolean
  Finite : Outport
  wires:
  Positions/1 -> Bus Selector/1
  Current Commands/1 -> Demux/1
  Bus Selector/1 -> Relational Operator/1  "<Motor A>"
  Bus Selector/2 -> Relational Operator1/1  "<Leg A>"
  Bus Selector/3 -> Relational Operator2/1  "<Motor B>"
  Bus Selector/4 -> Relational Operator3/1  "<Leg B>"
  Demux/1 -> Relational Operator4/1
  Demux/2 -> Relational Operator5/1
  Relational Operator/1 -> Logical Operator1/1
  Relational Operator1/1 -> Logical Operator1/2
  Relational Operator2/1 -> Logical Operator1/3
  Relational Operator3/1 -> Logical Operator1/4
  Relational Operator4/1 -> Logical Operator1/5
  Relational Operator5/1 -> Logical Operator1/6
  Logical Operator1/1 -> Finite/1

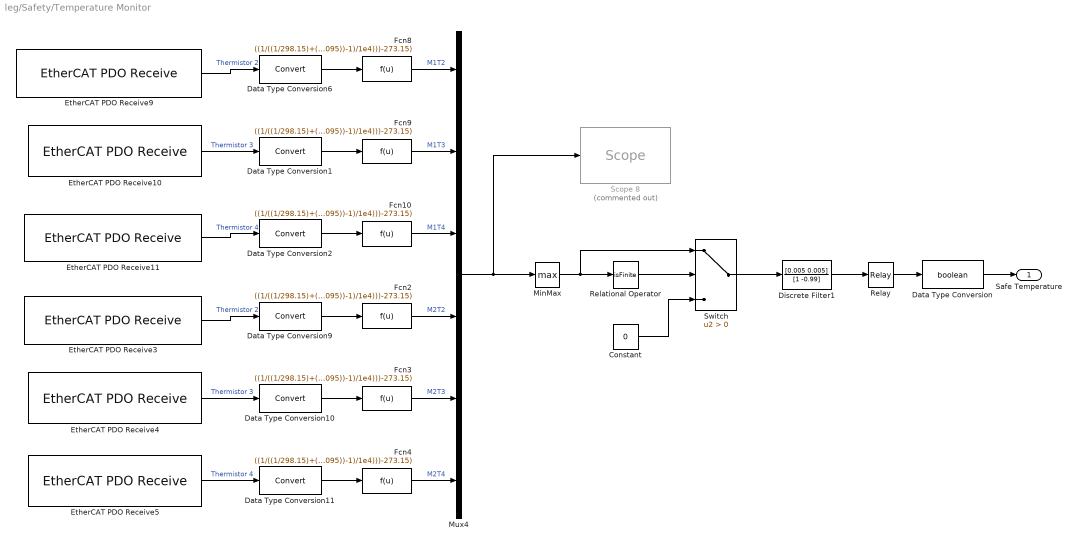
== system leg/Safety/Temperature Monitor ==
  Constant : Constant  Value=0
  Data Type Conversion : DataTypeConversion  OutDataTypeStr=boolean
  Data Type Conversion{1..2,6,9..11} (6 alike) : DataTypeConversion
  Discrete Filter1 : DiscreteFilter  Numerator=[0.005 0.005]  Denominator=[1 -0.99]  a0EqualsOne=on
  EtherCAT PDO Receive10 : xpcethercatlib/EtherCAT PDO Receive  Priority=2  sig_name=Box 4 (ATRIAS 2.1 Leg (Medulla 1.5)).Thermistors.Thermistor 3  sig_offset=1232  sig_type=uint16  type_size=16  sig_dim=1  device_id=0  sample_time=0.001000
  EtherCAT PDO Receive11 : xpcethercatlib/EtherCAT PDO Receive  Priority=2  sig_name=Box 4 (ATRIAS 2.1 Leg (Medulla 1.5)).Thermistors.Thermistor 4  sig_offset=1248  sig_type=uint16  type_size=16  sig_dim=1  device_id=0  sample_time=0.001000
  EtherCAT PDO Receive3 : xpcethercatlib/EtherCAT PDO Receive  Priority=2  sig_name=Box 3 (ATRIAS 2.1 Leg (Medulla 1.5)).Thermistors.Thermistor 2  sig_offset=840  sig_type=uint16  type_size=16  sig_dim=1  device_id=0  sample_time=0.001000
  EtherCAT PDO Receive4 : xpcethercatlib/EtherCAT PDO Receive  Priority=2  sig_name=Box 3 (ATRIAS 2.1 Leg (Medulla 1.5)).Thermistors.Thermistor 3  sig_offset=856  sig_type=uint16  type_size=16  sig_dim=1  device_id=0  sample_time=0.001000
  EtherCAT PDO Receive5 : xpcethercatlib/EtherCAT PDO Receive  Priority=2  sig_name=Box 3 (ATRIAS 2.1 Leg (Medulla 1.5)).Thermistors.Thermistor 4  sig_offset=872  sig_type=uint16  type_size=16  sig_dim=1  device_id=0  sample_time=0.001000
  EtherCAT PDO Receive9 : xpcethercatlib/EtherCAT PDO Receive  Priority=2  sig_name=Box 4 (ATRIAS 2.1 Leg (Medulla 1.5)).Thermistors.Thermistor 2  sig_offset=1216  sig_type=uint16  type_size=16  sig_dim=1  device_id=0  sample_time=0.001000
  Fcn{2..4,8..10} (6 alike) : Fcn  Expr=((1/((1/298.15)+(1/3988)*log(4700/((3.26/((u-172)*2.7/4095))-1)/1e4)))-273.15)
  MinMax : MinMax  Function=max
  Mux4 : Mux  Inputs=6
  Relational Operator : RelationalOperator  Operator=isFinite  OutDataTypeStr=boolean
  Relay : Relay  OnSwitchValue=80  OffSwitchValue=60  OnOutputValue=0  OffOutputValue=1
  Scope 8 : slrtlib/Displays and Logging/Scope   Commented=on  scopeno=4  scopetype=Target  autostart=on  viewmode=Numerical  formatstr='%15.6f'  grid=on  ylimits=[0,0]  nosamples=100  noprepostsamples=0  interleave=1  triggermode=FreeRun  triggersignal=1  trigsignalfromport=off  triggerlevel=0.0  triggerslope=Either  triggerscope=1  triggersample=0  filename=data.dat  mode=Lazy  writesize=512  autorestart=off  dynamicfilemode=off  maxwritefilesize=512*1024^2
  Switch : Switch  Criteria=u2 > Threshold
  Safe Temperature : Outport
  wires:
  EtherCAT PDO Receive5/1 -> Data Type Conversion11/1  "Thermistor 4"
  EtherCAT PDO Receive4/1 -> Data Type Conversion10/1  "Thermistor 3"
  EtherCAT PDO Receive3/1 -> Data Type Conversion9/1  "Thermistor 2"
  Mux4/1 -> Scope 8/1, MinMax/1
  Data Type Conversion11/1 -> Fcn4/1
  Data Type Conversion10/1 -> Fcn3/1
  Data Type Conversion9/1 -> Fcn2/1
  MinMax/1 -> Switch/1, Relational Operator/1
  Relational Operator/1 -> Switch/2
  Constant/1 -> Switch/3
  Switch/1 -> Discrete Filter1/1
  Discrete Filter1/1 -> Relay/1
  EtherCAT PDO Receive11/1 -> Data Type Conversion2/1  "Thermistor 4"
  EtherCAT PDO Receive10/1 -> Data Type Conversion1/1  "Thermistor 3"
  EtherCAT PDO Receive9/1 -> Data Type Conversion6/1  "Thermistor 2"
  Data Type Conversion2/1 -> Fcn10/1
  Data Type Conversion1/1 -> Fcn9/1
  Data Type Conversion6/1 -> Fcn8/1
  Fcn3/1 -> Mux4/5  "M2T3"
  Fcn2/1 -> Mux4/4  "M2T2"
  Fcn10/1 -> Mux4/3  "M1T4"
  Fcn8/1 -> Mux4/1  "M1T2"
  Fcn9/1 -> Mux4/2  "M1T3"
  Fcn4/1 -> Mux4/6  "M2T4"
  Relay/1 -> Data Type Conversion/1
  Data Type Conversion/1 -> Safe Temperature/1

== matlab function leg/Controller/MATLAB Function1 ==
  data: Fa2x input; Fas output; Fa2y input; th input; Fbs output
function [Fas, Fbs] = fcn(Fa2x, Fa2y, th)
%#codegen

L1 = 0.5;
L2 = 0.35;
Fas = (Fa2y*L1*cos(th) - Fa2x*L1*sin(th))/L2;
Fbs = -(Fa2y*L1)/L2;

== matlab function leg/Controller/MATLAB Function ==
  data: x input; y input; theta input; x1 output; y1 output
function [x1, y1] = rotate(x, y, theta)
%#codegen

v = [cos(theta), -sin(theta); sin(theta), cos(theta)]*[x; y];
x1 = v(1);
y1 = v(2);
